simulink model "LaserLight"  (R2017b)
settings: Solver=VariableStepAuto  StartTime=0.0  StopTime=1  RelTol=1e-3
values from neighbouring files (symbols this model uses):
  Amp0d = [255]    [System.m]
  Amp0n = [12]    [System.m]
  Amp1d = [255]    [System.m]
  Amp1n = [12]    [System.m]
  AmpSat0 = 12    [System.m]
  AmpSat1 = 12    [System.m]
  BackEMF0 = 0.001545    [System.m]
  BackEMF1 = 0.001545    [System.m]
  D = 10    [CONSTANTS.m]
  Elec0d = [.00105 2.25]    [System.m]
  Elec0n = [1]    [System.m]
  Elec1d = [1]    [0Controller.m]    (also in System.m = [.00105 2.25])
  Elec1n = [1]    [0Controller.m]    (also in System.m)
  FB1 = [1]    [0Controller.m]
  Mech0d = [1]    [0Controller.m]    (also in System.m = [0.000001283 0.00005157])
  Mech0n = [1]    [0Controller.m]    (also in System.m)
  Mech1d = [1]    [0Controller.m]    (also in System.m = [0.000001283 0.00005157])
  Mech1n = [1]    [0Controller.m]    (also in System.m)
  StFric0 = 0    [System.m]
  TConst0 = 0.0193    [System.m]
  TConst1 = 0.0193    [System.m]
undefined symbols (not defined in the file or in its folder): FB0
libraries: simulink x7
settings Model: Creator=Jimmy  LastModifiedBy=jmvsu
settings CodeAppCC: StateflowObjectComments=on

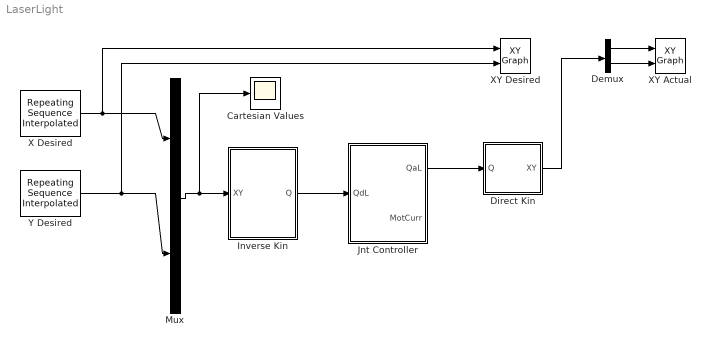
== system LaserLight ==
  Cartesian Values : Scope
  Demux : Demux  Outputs=2
  Direct Kin : Subsystem
  Inverse Kin : Subsystem
  Jnt Controller : Subsystem
  Mux : Mux  Inputs=2
  X Desired : simulink/Sources/Repeating Sequence Interpolated  OutValues=[100 100 -100 -100 100]  TimeValues=[0 0.25 0.5 0.75 1]  LookUpMeth=Interpolation-Use End Values  tsamp=0.01  OutMin=[]  OutMax=[]  OutDataTypeStr=double  OutputDataTypeScalingMode=double  OutDataType=fixdt(0,8)  OutScaling=2^-10
  XY Actual : simulink/Sinks/XY Graph  xmin=-125  xmax=125  ymin=-125  ymax=125  st=-1
  XY Desired : simulink/Sinks/XY Graph  xmin=-110  xmax=110  ymin=-110  ymax=110  st=-1
  Y Desired : simulink/Sources/Repeating Sequence Interpolated  OutValues=[-100 100 100 -100 -100]  TimeValues=[0 0.25 0.5 0.75 1]  LookUpMeth=Interpolation-Use End Values  tsamp=0.01  OutMin=[]  OutMax=[]  OutDataTypeStr=double  OutputDataTypeScalingMode=double  OutDataType=fixdt(0,8)  OutScaling=2^-10
  wires:
  Y Desired/1 -> XY Desired/2, Mux/2
  Demux/2 -> XY Actual/2
  Inverse Kin/1("Q ") -> Jnt Controller/1(QdL)
  Direct Kin/1(XY) -> Demux/1
  Jnt Controller/1(QaL) -> Direct Kin/1(Q)
  Demux/1 -> XY Actual/1
  Mux/1 -> Cartesian Values/1, Inverse Kin/1(XY)
  X Desired/1 -> Mux/1, XY Desired/1

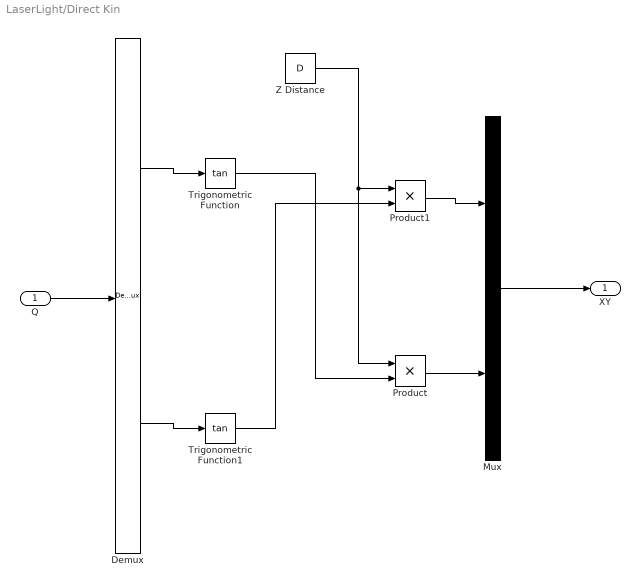
== system LaserLight/Direct Kin ==
  Q : Inport
  Demux : Demux  Outputs=2
  Mux : Mux  Inputs=2
  Product : Product
  Product1 : Product
  Trigonometric Function : Trigonometry  Operator=tan
  Trigonometric Function1 : Trigonometry  Operator=tan
  Z Distance : Constant  Value=D
  XY : Outport
  wires:
  Q/1 -> Demux/1
  Mux/1 -> XY/1
  Demux/1 -> Trigonometric Function/1
  Demux/2 -> Trigonometric Function1/1
  Trigonometric Function/1 -> Product/2
  Z Distance/1 -> Product1/1, Product/1
  Trigonometric Function1/1 -> Product1/2
  Product1/1 -> Mux/1
  Product/1 -> Mux/2

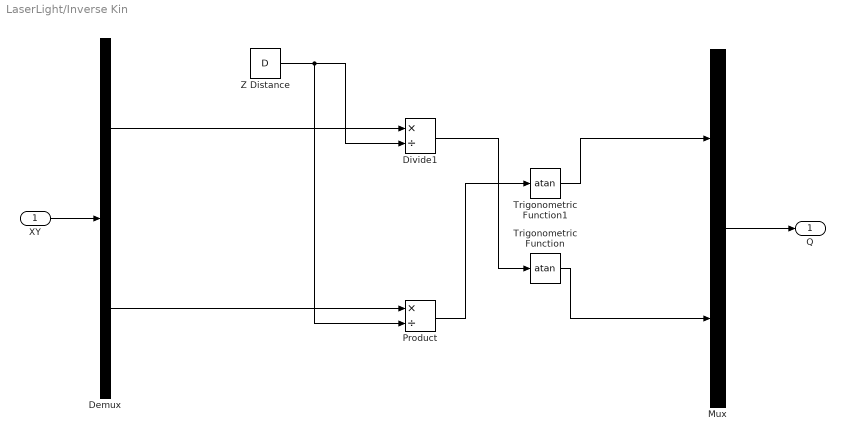
== system LaserLight/Inverse Kin ==
  XY : Inport
  Demux : Demux  Outputs=2
  Divide1 : Product  Inputs=*/
  Mux : Mux  Inputs=2
  Product : Product  Inputs=*/
  Trigonometric Function : Trigonometry  Operator=atan
  Trigonometric Function1 : Trigonometry  Operator=atan
  "Z Distance " : Constant  Value=D
  "Q " : Outport
  wires:
  XY/1 -> Demux/1
  Mux/1 -> "Q "/1
  Demux/1 -> Divide1/1
  Trigonometric Function/1 -> Mux/2
  Divide1/1 -> Trigonometric Function/1
  "Z Distance "/1 -> Product/2, Divide1/2
  Demux/2 -> Product/1
  Trigonometric Function1/1 -> Mux/1
  Product/1 -> Trigonometric Function1/1

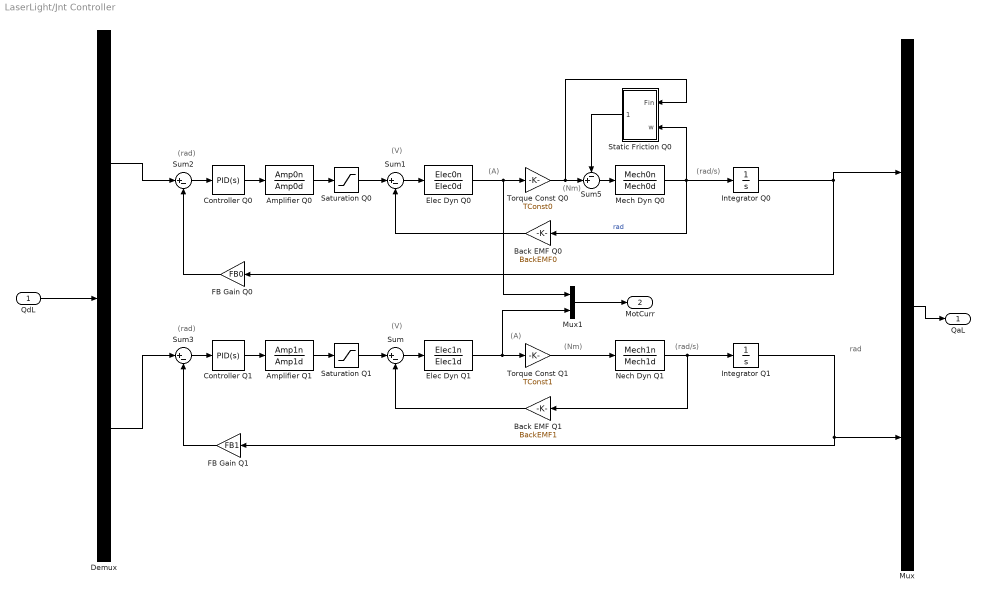
== system LaserLight/Jnt Controller ==
  note: rad
  note: (rad/s)
  note: (V)
  note: (rad)
  note: (rad/s)
  note: (A)
  note: (Nm)
  note: (V)
  note: (A)
  note: (rad)
  note: (Nm)
  QdL : Inport
  Amplifier Q0 : TransferFcn  Numerator=Amp0n  Denominator=Amp0d
  Amplifier Q1 : TransferFcn  Numerator=Amp1n  Denominator=Amp1d
  Back EMF Q0 : Gain  Gain=BackEMF0
  Back EMF Q1 : Gain  Gain=BackEMF1
  Controller Q0 : simulink/Continuous/PID Controller  Controller=PID  TimeDomain=Continuous-time  SampleTime=-1  IntegratorMethod=Forward Euler  FilterMethod=Forward Euler  Form=Parallel  UseFilter=on  ControllerParametersSource=internal  P=19.445961470142  I=200.878604706117  D=0.242603406733837  N=930.997703714061  InitialConditionSource=internal  InitialConditionForIntegrator=0  InitialConditionForFilter=0  ExternalReset=none  LimitOutput=off  UpperSaturationLimit=inf  LowerSaturationLimit=-inf  LinearizeAsGain=on  AntiWindupMode=none  Kb=1  TrackingMode=off  Kt=1  PParamMin=[]  PParamMax=[]  IParamMin=[]  IParamMax=[]  DParamMin=[]  DParamMax=[]  NParamMin=[]  NParamMax=[]  KbParamMin=[]  KbParamMax=[]  KtParamMin=[]  KtParamMax=[]  POutMin=[]  POutMax=[]  IOutMin=[]  IOutMax=[]  DOutMin=[]  DOutMax=[]  NOutMin=[]  NOutMax=[]  KbOutMin=[]  KbOutMax=[]  KtOutMin=[]  KtOutMax=[]  IntegratorOutMin=[]  IntegratorOutMax=[]  FilterOutMin=[]  FilterOutMax=[]  SumOutMin=[]  SumOutMax=[]  SumI1OutMin=[]  SumI1OutMax=[]  SumI2OutMin=[]  SumI2OutMax=[]  SumI3OutMin=[]  SumI3OutMax=[]  SumDOutMin=[]  SumDOutMax=[]  SaturationOutMin=[]  SaturationOutMax=[]  IntegratorContinuousStateAttributes=''  IntegratorStateMustResolveToSignalObject=off  IntegratorRTWStateStorageClass=Auto  FilterContinuousStateAttributes=''  FilterStateMustResolveToSignalObject=off  FilterRTWStateStorageClass=Auto  DifferentiatorICPrevScaledInput=0  DifferentiatorOutMin=[]  DifferentiatorOutMax=[]  InitialConditionSetting=State (most efficient)  FilterDiffOutCoefMin=[]  FilterDiffOutCoefMax=[]  SumDenOutMin=[]  SumDenOutMax=[]  SumNumOutMin=[]  SumNumOutMax=[]  ReciprocalOutMin=[]  ReciprocalOutMax=[]  DivideOutMin=[]  DivideOutMax=[]  TunerSelectOption=Transfer Function Based (PID Tuner App)
  Controller Q1 : simulink/Continuous/PID Controller  Controller=PID  TimeDomain=Continuous-time  SampleTime=-1  IntegratorMethod=Forward Euler  FilterMethod=Forward Euler  Form=Parallel  UseFilter=on  ControllerParametersSource=internal  P=19.445961470142  I=200.878604706117  D=0.242603406733837  N=930.997703714061  InitialConditionSource=internal  InitialConditionForIntegrator=0  InitialConditionForFilter=0  ExternalReset=none  LimitOutput=off  UpperSaturationLimit=inf  LowerSaturationLimit=-inf  LinearizeAsGain=on  AntiWindupMode=none  Kb=1  TrackingMode=off  Kt=1  PParamMin=[]  PParamMax=[]  IParamMin=[]  IParamMax=[]  DParamMin=[]  DParamMax=[]  NParamMin=[]  NParamMax=[]  KbParamMin=[]  KbParamMax=[]  KtParamMin=[]  KtParamMax=[]  POutMin=[]  POutMax=[]  IOutMin=[]  IOutMax=[]  DOutMin=[]  DOutMax=[]  NOutMin=[]  NOutMax=[]  KbOutMin=[]  KbOutMax=[]  KtOutMin=[]  KtOutMax=[]  IntegratorOutMin=[]  IntegratorOutMax=[]  FilterOutMin=[]  FilterOutMax=[]  SumOutMin=[]  SumOutMax=[]  SumI1OutMin=[]  SumI1OutMax=[]  SumI2OutMin=[]  SumI2OutMax=[]  SumI3OutMin=[]  SumI3OutMax=[]  SumDOutMin=[]  SumDOutMax=[]  SaturationOutMin=[]  SaturationOutMax=[]  IntegratorContinuousStateAttributes=''  IntegratorStateMustResolveToSignalObject=off  IntegratorRTWStateStorageClass=Auto  FilterContinuousStateAttributes=''  FilterStateMustResolveToSignalObject=off  FilterRTWStateStorageClass=Auto  DifferentiatorICPrevScaledInput=0  DifferentiatorOutMin=[]  DifferentiatorOutMax=[]  InitialConditionSetting=State (most efficient)  FilterDiffOutCoefMin=[]  FilterDiffOutCoefMax=[]  SumDenOutMin=[]  SumDenOutMax=[]  SumNumOutMin=[]  SumNumOutMax=[]  ReciprocalOutMin=[]  ReciprocalOutMax=[]  DivideOutMin=[]  DivideOutMax=[]  TunerSelectOption=Transfer Function Based (PID Tuner App)
  Demux : Demux  Outputs=2
  Elec Dyn Q0 : TransferFcn  Numerator=Elec0n  Denominator=Elec0d
  Elec Dyn Q1 : TransferFcn  Numerator=Elec1n  Denominator=Elec1d
  FB Gain Q0 : Gain  Gain=FB0
  FB Gain Q1 : Gain  Gain=FB1
  Integrator Q0 : Integrator
  Integrator Q1 : Integrator
  Mech Dyn Q0 : TransferFcn  Numerator=Mech0n  Denominator=Mech0d
  Mux : Mux  Inputs=2
  Mux1 : Mux  Inputs=2
  Nech Dyn Q1 : TransferFcn  Numerator=Mech1n  Denominator=Mech1d
  Saturation Q0 : Saturate  UpperLimit=AmpSat0  LowerLimit=-AmpSat0
  Saturation Q1 : Saturate  UpperLimit=AmpSat1  LowerLimit=-AmpSat1
  Static Friction Q0 : Subsystem
  Sum{,1..3} (4 alike) : Sum  Inputs=|+-
  Sum5 : Sum  Inputs=-+|
  Torque Const Q0 : Gain  Gain=TConst0
  Torque Const Q1 : Gain  Gain=TConst1
  QaL : Outport
  MotCurr : Outport  Port=2
  wires:
  QdL/1 -> Demux/1
  Mux/1 -> QaL/1
  Elec Dyn Q0/1 -> Torque Const Q0/1, Mux1/1
  Nech Dyn Q1/1 -> Integrator Q1/1, Back EMF Q1/1
  Sum/1 -> Elec Dyn Q1/1
  Torque Const Q0/1 -> Static Friction Q0/1(Fin), Sum5/2
  Mech Dyn Q0/1 -> Static Friction Q0/2(w), Integrator Q0/1, Back EMF Q0/1  "rad"
  FB Gain Q0/1 -> Sum2/2
  Mux1/1 -> MotCurr/1
  Sum3/1 -> Controller Q1/1
  Static Friction Q0/1(Fout) -> Sum5/1
  Torque Const Q1/1 -> Nech Dyn Q1/1
  FB Gain Q1/1 -> Sum3/2
  Amplifier Q1/1 -> Saturation Q1/1
  Sum1/1 -> Elec Dyn Q0/1
  Demux/2 -> Sum3/1
  Back EMF Q0/1 -> Sum1/2
  Integrator Q1/1 -> FB Gain Q1/1, Mux/2
  Saturation Q1/1 -> Sum/1
  Sum5/1 -> Mech Dyn Q0/1
  Back EMF Q1/1 -> Sum/2
  Controller Q0/1 -> Amplifier Q0/1
  Elec Dyn Q1/1 -> Mux1/2, Torque Const Q1/1
  Demux/1 -> Sum2/1
  Integrator Q0/1 -> FB Gain Q0/1, Mux/1
  Controller Q1/1 -> Amplifier Q1/1
  Amplifier Q0/1 -> Saturation Q0/1
  Sum2/1 -> Controller Q0/1
  Saturation Q0/1 -> Sum1/1

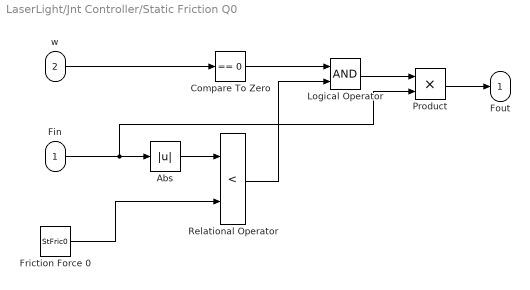
== system LaserLight/Jnt Controller/Static Friction Q0 ==
  Fin : Inport
  w : Inport  Port=2
  Abs : Abs
  Compare To Zero : simulink/Logic and Bit Operations/Compare To Zero  relop===  OutDataTypeStr=boolean
  Friction Force 0 : Constant  Value=StFric0
  Logical Operator : Logic  AllPortsSameDT=off  OutDataTypeStr=boolean
  Product : Product
  Relational Operator : RelationalOperator  Operator=<  OutDataTypeStr=boolean  RndMeth=Simplest
  Fout : Outport
  wires:
  Friction Force 0/1 -> Relational Operator/2
  Product/1 -> Fout/1
  Compare To Zero/1 -> Logical Operator/1
  Relational Operator/1 -> Logical Operator/2
  Logical Operator/1 -> Product/1
  Fin/1 -> Product/2, Abs/1
  w/1 -> Compare To Zero/1
  Abs/1 -> Relational Operator/1
